simulink model "paramdJdq"  (Simulink 8.3)
settings: Solver=ode45  StartTime=0.0  StopTime=10.0  RelTol=1e-3
libraries: WBCLibrary x7
settings Model: Creator=jorhabib  LastModifiedBy=jorhabib
settings DataIOCC: SignalLoggingSaveFormat=Dataset
settings DebuggingCC: UnderspecifiedInitializationDetection=Simplified  StateNameClashWarn=none
settings GRTTargetCC: CombineOutputUpdateFcns=on  GRTInterface=off

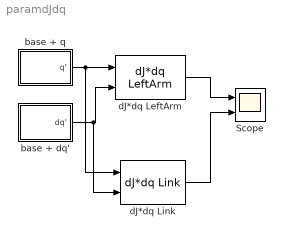
== system paramdJdq ==
  Scope : Scope  NumInputPorts=2
      settings: ShowLegends=on  YMin=-5~-5  YMax=5~5
  base + dq' : Subsystem
  base + q : Subsystem
  dJ*dq LeftArm : WBCLibrary/wholeBodyModel/Dynamics/dJ*dq LeftArm  val=9  robotName=robotName  localName=localName
  dJ*dq Link : WBCLibrary/wholeBodyModel/Dynamics/dJ*dq Link  val=19  robotName=robotName  localName=localName  link=l_gripper
  wires:
  base + q/1(q') -> dJ*dq Link/1, dJ*dq LeftArm/1
  base + dq'/1(dq') -> dJ*dq Link/2, dJ*dq LeftArm/2
  dJ*dq LeftArm/1 -> Scope/1
  dJ*dq Link/1 -> Scope/2

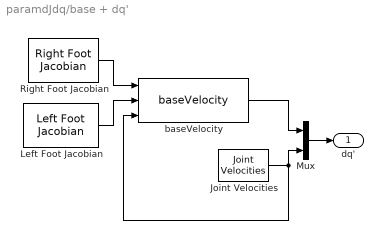
== system paramdJdq/base + dq' ==
  Joint Velocities : WBCLibrary/wholeBodyStates/Joint Velocities  robotName=robotName  localName=localName
  Left Foot Jacobian : WBCLibrary/wholeBodyModel/Jacobians/Left Foot Jacobian  robotName=robotName  localName=localName
  Mux : Mux  Inputs=2
  Right Foot Jacobian : WBCLibrary/wholeBodyModel/Jacobians/Right Foot Jacobian  robotName=robotName  localName=localName
  baseVelocity : WBCLibrary/Utilities/baseVelocity
  dq' : Outport
  wires:
  Left Foot Jacobian/1 -> baseVelocity/2
  Right Foot Jacobian/1 -> baseVelocity/1
  baseVelocity/1 -> Mux/1
  Joint Velocities/1 -> baseVelocity/3, Mux/2
  Mux/1 -> dq'/1

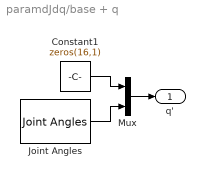
== system paramdJdq/base + q ==
  Constant1 : Constant  Value=zeros(16,1)
  Joint Angles : WBCLibrary/wholeBodyStates/Joint Angles  robotName=robotName  localName=localName
  Mux : Mux  Inputs=2
  q' : Outport
  wires:
  Mux/1 -> q'/1
  Joint Angles/1 -> Mux/2
  Constant1/1 -> Mux/1
